simulink model "Car_Model_PT_Project_Feedback_Manuscript"  (R2025b)
settings: Solver=VariableStepAuto  StartTime=0.0  StopTime=3000  FixedStep=1  MaxStep=0.001  RelTol=1e-6
libraries: SignalEditorBlockLib x2, simulink x1
settings Model: Creator=S25145249
settings SolverCC: ZeroCrossAlgorithm=Adaptive
settings DebuggingCC: IgnoredZcDiagnostic=none

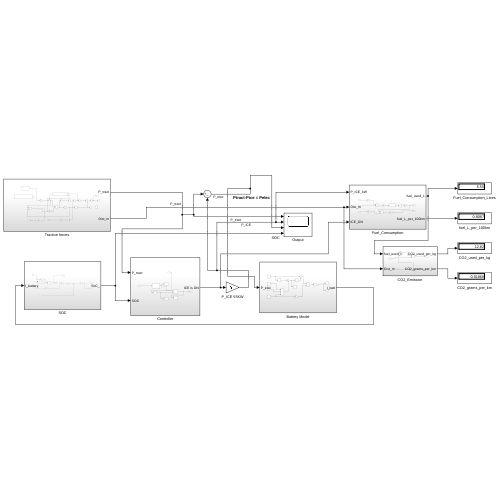
[thumbnail: Simulink's stored preview of the top-level diagram]
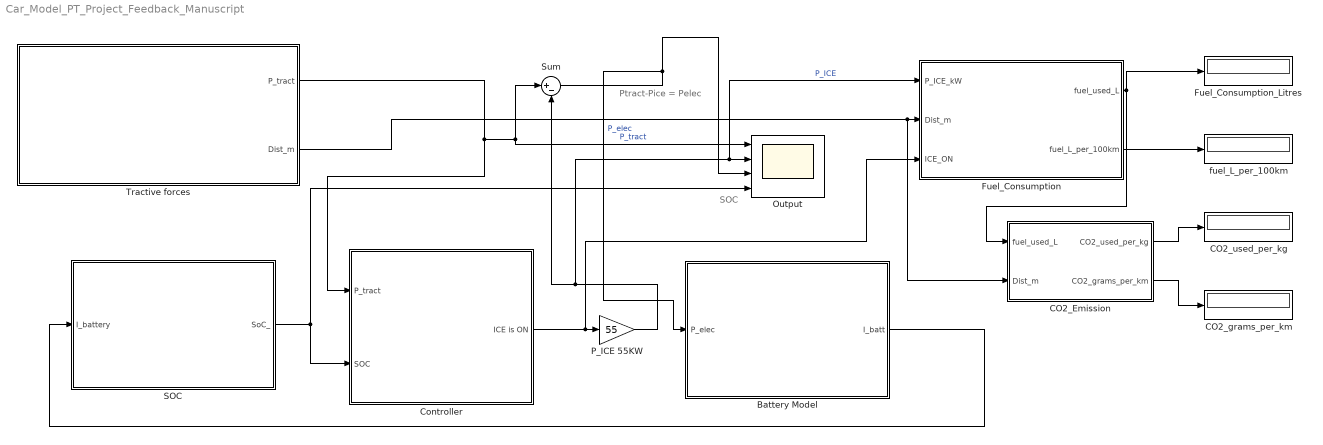
== system Car_Model_PT_Project_Feedback_Manuscript ==
  note: Ptract-Pice = Pelec
  note: SOC
  Battery Model : Subsystem
  CO2_Emission : Subsystem
  CO2_grams_per_km : Display
  CO2_used_per_kg : Display
  Controller : Subsystem
  Fuel_Consumption : Subsystem
  Fuel_Consumption_Litres : Display
  Output : Scope  NumInputPorts=4
      settings: ActiveDisplayYMinimum=-64.062897072548139  ActiveDisplayYMaximum=103.40655990798206  DataLoggingVariableName=ScopeData4
  P_ICE 55KW : Gain  Gain=55
  SOC : Subsystem
  Sum : Sum  Inputs=|+-
  Tractive forces : Subsystem
  fuel_L_per_100km : Display
  wires:
  SOC/1(SoC_) -> Output/4, Controller/2(SOC)
  Tractive forces/1(P_tract) -> Controller/1(P_tract), Sum/1, Output/1  "P_tract"
  P_ICE 55KW/1 -> Sum/2, Output/2, Fuel_Consumption/1(P_ICE_kW)  "P_ICE"
  Battery Model/1(I_batt) -> SOC/1(I_battery)
  Controller/1(ICE is ON) -> Fuel_Consumption/3(ICE_ON), P_ICE 55KW/1
  Tractive forces/2(Dist_m) -> CO2_Emission/2(Dist_m), Fuel_Consumption/2(Dist_m)
  Fuel_Consumption/1(fuel_used_L) -> Fuel_Consumption_Litres/1, CO2_Emission/1(fuel_used_L)
  Sum/1 -> Output/3, Battery Model/1(P_elec)  "P_elec"
  CO2_Emission/1(CO2_used_per_kg) -> CO2_used_per_kg/1
  Fuel_Consumption/2(fuel_L_per_100km) -> fuel_L_per_100km/1
  CO2_Emission/2(CO2_grams_per_km) -> CO2_grams_per_km/1

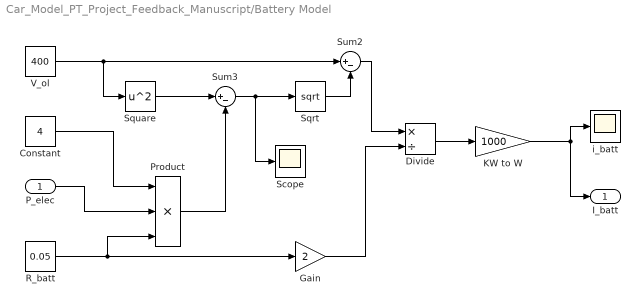
== system Car_Model_PT_Project_Feedback_Manuscript/Battery Model ==
  P_elec : Inport
  Constant : Constant  Value=4
  Divide : Product  Inputs=*/
  Gain : Gain  Gain=2
  KW to W : Gain  Gain=1000
  Product : Product  Inputs=3
  R_batt : Constant  Value=0.05
  Scope : Scope
      settings: ActiveDisplayYMinimum=159994.60479  ActiveDisplayYMaximum=160018.37725  DataLoggingVariableName=ScopeData5
  Sqrt : Sqrt
  Square : Math  Operator=square
  Sum2 : Sum  Inputs=|+-
  Sum3 : Sum  Inputs=|+-
  V_ol : Constant  Value=400
  i_batt : Scope
      settings: ActiveDisplayYMinimum=-114.85498  ActiveDisplayYMaximum=33.71985  DataLoggingVariableName=ScopeData3
  I_batt : Outport
  wires:
  Divide/1 -> KW to W/1
  Constant/1 -> Product/1
  R_batt/1 -> Gain/1, Product/3
  Sqrt/1 -> Sum2/2
  Square/1 -> Sum3/1
  Sum2/1 -> Divide/1
  Gain/1 -> Divide/2
  V_ol/1 -> Square/1, Sum2/1
  Sum3/1 -> Sqrt/1, Scope/1
  Product/1 -> Sum3/2
  P_elec/1 -> Product/2
  KW to W/1 -> I_batt/1, i_batt/1

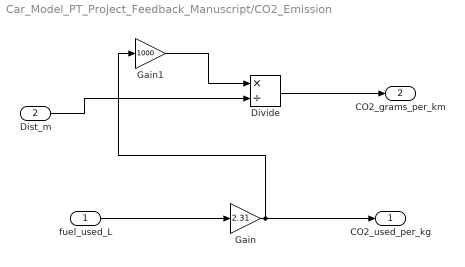
== system Car_Model_PT_Project_Feedback_Manuscript/CO2_Emission ==
  fuel_used_L : Inport
  Dist_m : Inport  Port=2
  Divide : Product  Inputs=*/
  Gain : Gain  Gain=2.31
  Gain1 : Gain  Gain=1000
  CO2_used_per_kg : Outport
  CO2_grams_per_km : Outport  Port=2  VectorParamsAs1DForOutWhenUnconnected=off
  wires:
  fuel_used_L/1 -> Gain/1
  Gain/1 -> Gain1/1, CO2_used_per_kg/1
  Gain1/1 -> Divide/1
  Dist_m/1 -> Divide/2
  Divide/1 -> CO2_grams_per_km/1

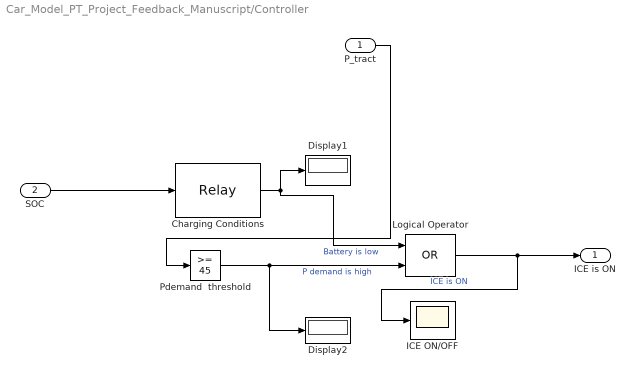
== system Car_Model_PT_Project_Feedback_Manuscript/Controller ==
  P_tract : Inport
  SOC : Inport  Port=2
  Charging Conditions : Relay  OnSwitchValue=75  OffSwitchValue=30  OnOutputValue=0  OffOutputValue=1
  Display1 : Display
  Display2 : Display
  ICE ON/OFF : Scope
      settings: ActiveDisplayYMinimum=-0.125  ActiveDisplayYMaximum=1.125
  Logical Operator : Logic  Operator=OR  AllPortsSameDT=off  OutDataTypeStr=boolean
  Pdemand  threshold : simulink/Logic and Bit Operations/Compare To Constant  relop=>=  const=45  OutDataTypeStr=boolean
  ICE is ON : Outport
  wires:
  SOC/1 -> Charging Conditions/1
  P_tract/1 -> Pdemand  threshold/1
  Charging Conditions/1 -> Logical Operator/1, Display1/1  "Battery is low"
  Pdemand  threshold/1 -> Display2/1, Logical Operator/2  "P demand is high"
  Logical Operator/1 -> ICE is ON/1, ICE ON/OFF/1  "ICE is ON"

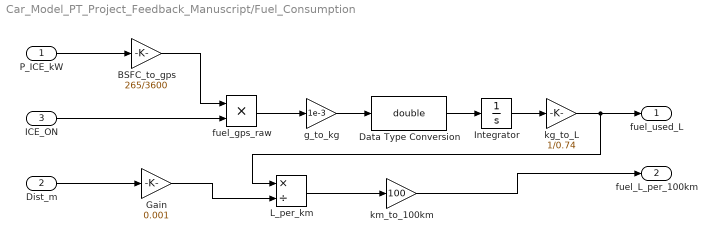
== system Car_Model_PT_Project_Feedback_Manuscript/Fuel_Consumption ==
  P_ICE_kW : Inport
  Dist_m : Inport  Port=2
  ICE_ON : Inport  Port=3
  BSFC_to_gps : Gain  Gain=265/3600
  Data Type Conversion : DataTypeConversion  OutDataTypeStr=double  SaturateOnIntegerOverflow=off  RndMeth=Floor
  Gain : Gain  Gain=0.001
  Integrator : Integrator
  L_per_km : Product  Inputs=*/
  fuel_gps_raw : Product
  g_to_kg : Gain  Gain=1e-3
  kg_to_L : Gain  Gain=1/0.74
  km_to_100km : Gain  Gain=100
  fuel_used_L : Outport
  fuel_L_per_100km : Outport  Port=2
  wires:
  P_ICE_kW/1 -> BSFC_to_gps/1
  BSFC_to_gps/1 -> fuel_gps_raw/1
  ICE_ON/1 -> fuel_gps_raw/2
  fuel_gps_raw/1 -> g_to_kg/1
  g_to_kg/1 -> Data Type Conversion/1
  Integrator/1 -> kg_to_L/1
  kg_to_L/1 -> L_per_km/1, fuel_used_L/1
  Dist_m/1 -> Gain/1
  Gain/1 -> L_per_km/2
  L_per_km/1 -> km_to_100km/1
  km_to_100km/1 -> fuel_L_per_100km/1
  Data Type Conversion/1 -> Integrator/1

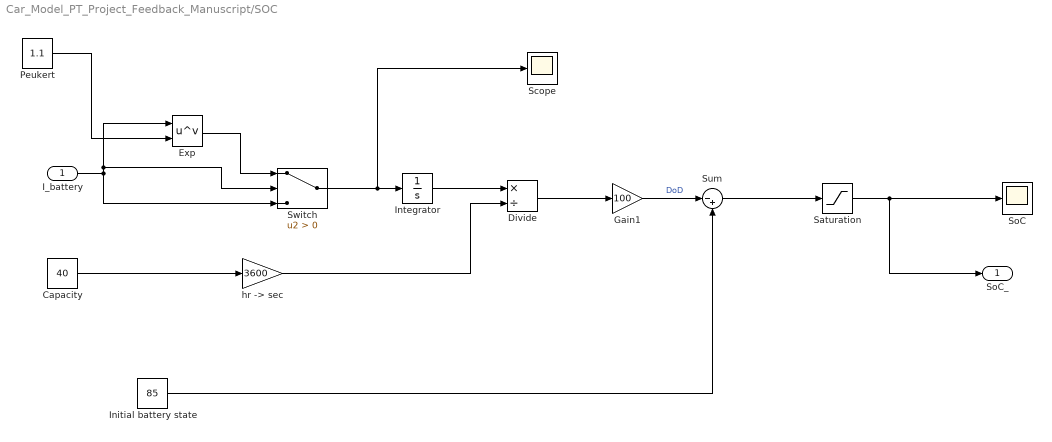
== system Car_Model_PT_Project_Feedback_Manuscript/SOC ==
  I_battery : Inport
  Capacity : Constant  Value=40
  Divide : Product  Inputs=*/
  Exp : Math  Operator=pow
  Gain1 : Gain  Gain=100
  Initial battery state : Constant  Value=85
  Integrator : Integrator
  Peukert : Constant  Value=1.1
  Saturation : Saturate  UpperLimit=100  LowerLimit=0
  Scope : Scope
      settings: ActiveDisplayYMinimum=-115.65994  ActiveDisplayYMaximum=40.9645  DataLoggingVariableName=ScopeData4
  SoC : Scope
      settings: ActiveDisplayYMinimum=1.25  ActiveDisplayYMaximum=88.75
  Sum : Sum  Inputs=|-+
  Switch : Switch  Criteria=u2 > Threshold  SaturateOnIntegerOverflow=off  InputSameDT=off
  "hr -> sec" : Gain  Gain=3600
  SoC_ : Outport
  wires:
  I_battery/1 -> Exp/1, Switch/2, Switch/3
  "hr -> sec"/1 -> Divide/2
  Divide/1 -> Gain1/1
  Capacity/1 -> "hr -> sec"/1
  Gain1/1 -> Sum/1  "DoD"
  Peukert/1 -> Exp/2
  Switch/1 -> Scope/1, Integrator/1
  Exp/1 -> Switch/1
  Integrator/1 -> Divide/1
  Saturation/1 -> SoC_/1, SoC/1
  Initial battery state/1 -> Sum/2
  Sum/1 -> Saturation/1

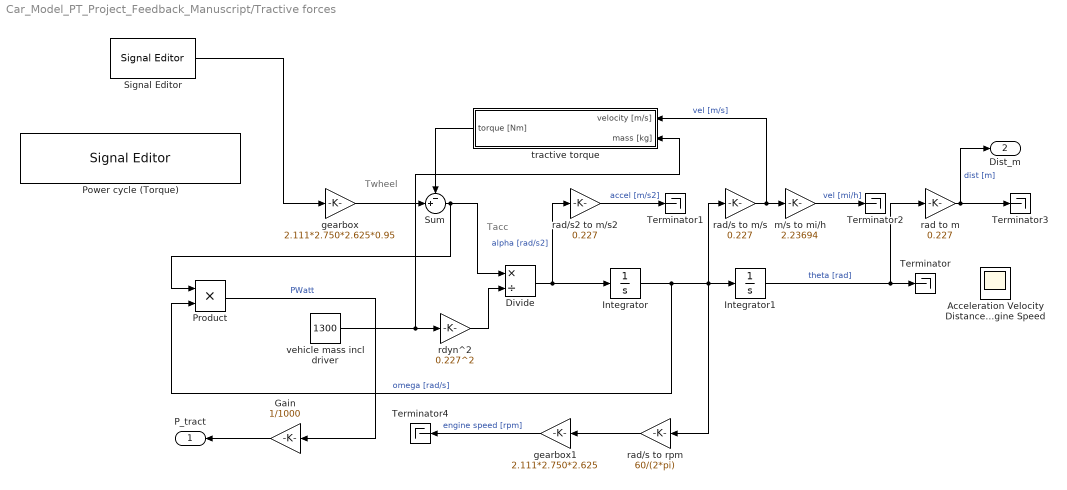
== system Car_Model_PT_Project_Feedback_Manuscript/Tractive forces ==
  note: Tacc
  note: Twheel
  Acceleration Velocity Distance Engine Speed : Scope
      settings: IsFloating=on  Floating=on  ActiveDisplayYMinimum=5.6184823541906912  ActiveDisplayYMaximum=6.2437947592259979
  Divide : Product  Inputs=*/
  Gain : Gain  Gain=1/1000
  Integrator : Integrator
  Integrator1 : Integrator
  Power cycle (Torque) : SignalEditorBlockLib/Signal Editor  FileName=Power_cycle120.mat  ActiveScenario=Scenario  ActiveSignal=Signal 1  IsBus=off  OutputBusObjectStr=Bus: BusObject  SampleTime=0  ZeroCross=off  OutputAfterFinalValue=Setting to zero  Unit=inherit  PreserveSignalName=on  ApplySigPropsToAllScenarios=on  ApplySigPropsToAllSignals=off  SignalPropertySource=Dialog parameters
  Product : Product
  Signal Editor : SignalEditorBlockLib/Signal Editor  FileName=feedback.mat  ActiveScenario=Scenario  ActiveSignal=Signal 1  IsBus=off  OutputBusObjectStr=Bus: BusObject  SampleTime=0  ZeroCross=off  OutputAfterFinalValue=Setting to zero  Unit=inherit  PreserveSignalName=on  ApplySigPropsToAllScenarios=on  ApplySigPropsToAllSignals=off  SignalPropertySource=Dialog parameters
  Sum : Sum  Inputs=-+|
  Terminator{,1..4} (5 alike) : Terminator
  gearbox : Gain  Gain=2.111*2.750*2.625*0.95
  gearbox1 : Gain  Gain=2.111*2.750*2.625
  m/s to mi/h : Gain  Gain=2.23694
  rad to m : Gain  Gain=0.227
  rad/s to m/s : Gain  Gain=0.227
  rad/s to rpm : Gain  Gain=60/(2*pi)
  rad/s2 to m/s2 : Gain  Gain=0.227
  rdyn^2 : Gain  Gain=0.227^2
  tractive torque : Subsystem
  vehicle mass incl driver : Constant  Value=1300
  P_tract : Outport
  Dist_m : Outport  Port=2  VectorParamsAs1DForOutWhenUnconnected=off
  wires:
  rad to m/1 -> Dist_m/1, Terminator3/1  "dist [m]"
  rad/s to rpm/1 -> gearbox1/1
  gearbox/1 -> Sum/2
  Integrator1/1 -> Terminator/1, rad to m/1  "theta [rad]"
  Sum/1 -> Product/1, Divide/1
  Integrator/1 -> Product/2, rad/s to rpm/1, rad/s to m/s/1, Integrator1/1  "omega [rad/s]"
  rad/s to m/s/1 -> m/s to mi/h/1, tractive torque/1(velocity [m/s])  "vel [m/s]"
  rad/s2 to m/s2/1 -> Terminator1/1  "accel [m/s2]"
  m/s to mi/h/1 -> Terminator2/1  "vel [mi/h]"
  tractive torque/1(torque [Nm]) -> Sum/1
  gearbox1/1 -> Terminator4/1  "engine speed [rpm]"
  rdyn^2/1 -> Divide/2
  vehicle mass incl driver/1 -> rdyn^2/1, tractive torque/2(mass [kg])
  Divide/1 -> Integrator/1, rad/s2 to m/s2/1  "alpha [rad/s2]"
  Product/1 -> Gain/1  "PWatt"
  Gain/1 -> P_tract/1
  Signal Editor/1 -> gearbox/1

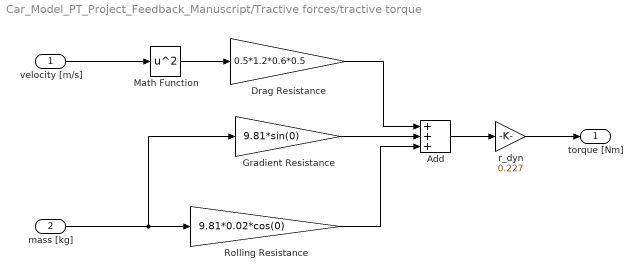
== system Car_Model_PT_Project_Feedback_Manuscript/Tractive forces/tractive torque ==
  velocity [m/s] : Inport
  mass [kg] : Inport  Port=2
  Add : Sum  Inputs=+++
  Drag Resistance : Gain  Gain=0.5*1.2*0.6*0.5
  Gradient Resistance : Gain  Gain=9.81*sin(0)
  Math Function : Math  Operator=square  SignedPower=on
  Rolling Resistance : Gain  Gain=9.81*0.02*cos(0)
  r_dyn : Gain  Gain=0.227
  torque [Nm] : Outport  VectorParamsAs1DForOutWhenUnconnected=off
  wires:
  r_dyn/1 -> torque [Nm]/1
  velocity [m/s]/1 -> Math Function/1
  Math Function/1 -> Drag Resistance/1
  Add/1 -> r_dyn/1
  Drag Resistance/1 -> Add/1
  Gradient Resistance/1 -> Add/2
  Rolling Resistance/1 -> Add/3
  mass [kg]/1 -> Rolling Resistance/1, Gradient Resistance/1
